simulink model "ControlMRAC"  (R2022b)
settings: Solver=VariableStepAuto  StartTime=0.0  StopTime=10.0  RelTol=1e-3
undefined symbols (not defined in the file): A, B, Psi1, Psi2, V0, W1, W2
settings Model: Creator=raul  LastModifiedBy=raul

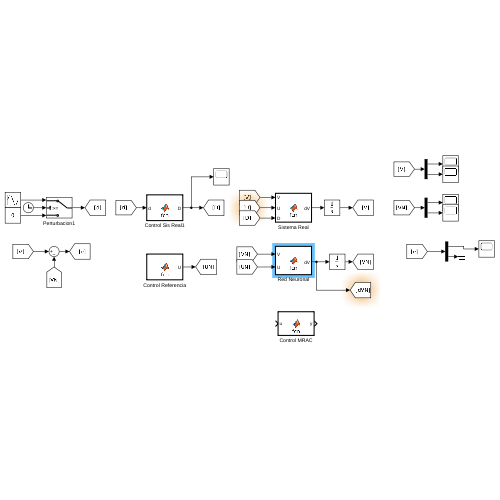
[thumbnail: Simulink's stored preview of the top-level diagram]
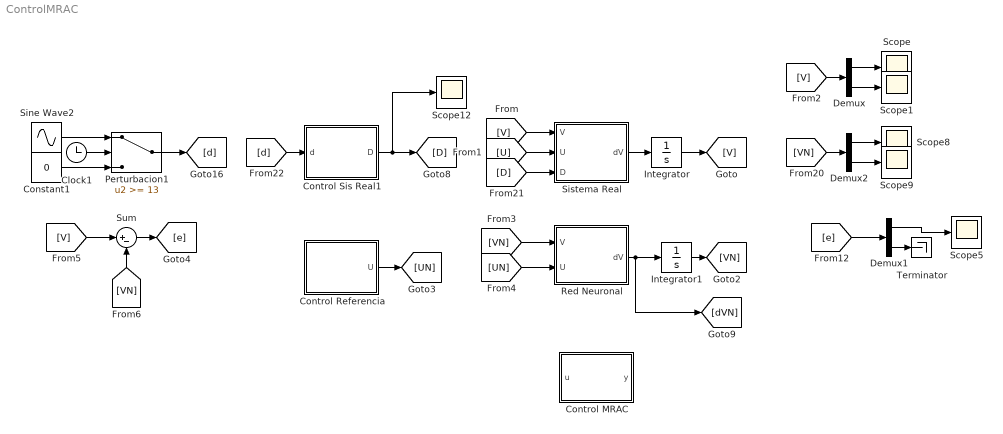
== system ControlMRAC ==
  Clock1 : Clock
  Constant1 : Constant  Value=0
  Control MRAC : MATLAB Function  TreatAsAtomicUnit=on
  Control Referencia : MATLAB Function  TreatAsAtomicUnit=on
  Control Sis Real1 : MATLAB Function  TreatAsAtomicUnit=on
  Demux : Demux  Outputs=2
  Demux1 : Demux  Outputs=2
  Demux2 : Demux  Outputs=2
  Integrator : Integrator  InitialCondition=V0
  Integrator1 : Integrator  InitialCondition=V0
  Perturbacion1 : Switch  Threshold=13  SaturateOnIntegerOverflow=off  InputSameDT=off
  Red Neuronal : MATLAB Function  TreatAsAtomicUnit=on
  Scope{,1,5,8..9,12} (6 alike) : Scope
  Sine Wave2 : Sin  Frequency=5  SampleTime=0
  Sistema Real : MATLAB Function  TreatAsAtomicUnit=on
  Sum : Sum  Inputs=|+-
  Terminator : Terminator
  wires:
  [V] -> Demux/1
  Demux/1 -> Scope/1
  [d] -> Control Sis Real1/1(d)
  [V] -> Sistema Real/1(V)
  Integrator/1 -> [V]
  Sistema Real/1(dV) -> Integrator/1
  [U] -> Sistema Real/2(U)
  [VN] -> Demux2/1
  Demux2/2 -> Scope9/1
  Control Sis Real1/1(D) -> Scope12/1, [D]
  [D] -> Sistema Real/3(D)
  Demux/2 -> Scope1/1
  Demux2/1 -> Scope8/1
  Perturbacion1/1 -> [d]
  Sine Wave2/1 -> Perturbacion1/1
  Clock1/1 -> Perturbacion1/2
  Constant1/1 -> Perturbacion1/3
  Sum/1 -> [e]
  [V] -> Sum/1
  [VN] -> Sum/2
  [e] -> Demux1/1
  Demux1/1 -> Scope5/1
  Demux1/2 -> Terminator/1
  Control Referencia/1(U) -> [UN]
  [UN] -> Red Neuronal/2(U)
  Integrator1/1 -> [VN]
  Red Neuronal/1(dV) -> [dVN], Integrator1/1
  [VN] -> Red Neuronal/1(V)

== matlab function ControlMRAC/Control MRAC ==
  data: u input; y output
function y = fcn(u)

y = u;

== matlab function ControlMRAC/Sistema Real ==
  data: V input; U input; dV output; W1 parameter; W2 parameter; Psi1 parameter; Psi2 parameter; B parameter; A parameter; D input
function dV  = fcn(V, U, W1, W2, Psi1, Psi2, B, A,D)

dV=A*V+B*(W1*sigmoid(Psi1,V)+W2*phi_sigmoid(Psi2,V)*U+W2*phi_sigmoid(Psi2,V)*D);


function s = sigmoid(b,x)
   s = 1./(1+exp(-b*x)); 
end



function phi = phi_sigmoid(bp, xp)
    % Comprueba que b y x tengan las dimensiones adecuadas
    [rows_b, cols_b] = size(bp);
%     [rows_x, cols_x] = size(xp);

    % Inicializa la matriz de salida
    phi = zeros(rows_b, rows_b); % Matriz de 20x20

    % Calcula la sigmoide combinando cada fila de b con el vector x
    for i = 1:rows_b
        phi(i, :) = 1 ./ (1 + exp(-bp(i, :) * xp)); % Producto y sigmoide
    end
end



end

== matlab function ControlMRAC/Red Neuronal ==
  data: V input; U input; dV output; W1 parameter; W2 parameter; Psi1 parameter; Psi2 parameter; B parameter; A parameter
function dV  = fcn(V, U, W1, W2, Psi1, Psi2, B, A)

dV=A*V+B*(W1*sigmoid(Psi1,V)+W2*phi_sigmoid(Psi2,V)*U);


function s = sigmoid(b,x)
   s = 1./(1+exp(-b*x)); 
end



function phi = phi_sigmoid(bp, xp)
    % Comprueba que b y x tengan las dimensiones adecuadas
    [rows_b, cols_b] = size(bp);
%     [rows_x, cols_x] = size(xp);

    % Inicializa la matriz de salida
    phi = zeros(rows_b, rows_b); % Matriz de 20x20

    % Calcula la sigmoide combinando cada fila de b con el vector x
    for i = 1:rows_b
        phi(i, :) = 1 ./ (1 + exp(-bp(i, :) * xp)); % Producto y sigmoide
    end
end



end

== matlab function ControlMRAC/Control Referencia ==
  data: U output
function U = fcn()%add Bw,w

U=zeros(20,1);

== matlab function ControlMRAC/Control Sis Real1 ==
  data: D output; d input; nodeDisturbe parameter
function D = fcn(d, nodeDisturbe)%add Bw,w

D=zeros(20,1);
D(nodeDisturbe,1)=d;
